simulink library "libFlightGearAnimation"  (R2020b)
settings: Solver=VariableStepAuto  StartTime=0.0  StopTime=10.0  RelTol=1e-3
undefined symbols (not defined in the file): outputs, Receive, Send, stepTime
libraries: aerolibconvert2 x3, aerolibfltsims x3, aerolibanimutils x1
settings Model: Creator=caatay  LastModifiedBy=caatay

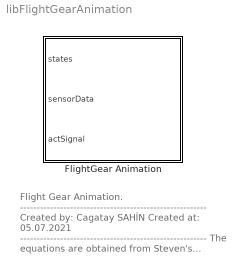
== system libFlightGearAnimation ==
  note: Flight Gear Animation.
      | --------------------------------------------------------
      | Created by: Cagatay SAHİN
      | Created at: 05.07.2021
      | --------------------------------------------------------
      | The equations are obtained from
      | Steven's textbook.
      | The reference book can be found in
      | "references folder".
      | --------------------------------------------------------
      | for question:
      | cagataysahin44@gmail.com
  FlightGear Animation : Subsystem  mask(Animation Model - Flight Gear Animation Model){stepTime=stepTime}
      mask prompts: stepTime "Step Sİze for each Step"
      mask help: Animation of aircraft's at whole simulation. That block use, states sensor data, actuator signals.
      mask Help:
      | This block is used for animate aircraft's motion in whole simulation.
      | --------------------------------------------------------------------------------------------------------------------------------------------------
      | Input of the function:
      | 	states: State Information
      | 	Sensor Data: Sensor Information.
      | 	Actuator Signal: Actuator Information
      | --------------------------------------------------------------------------------------------------------------------------------------------------
      | for question: "cagataysahin44@gmail.com"
      mask Display:
      | port_label('input',1,'states','texmode','on');
      | port_label('input',2,'sensorData','texmode','on');
      | port_label('input',3,'actSignal','texmode','on');

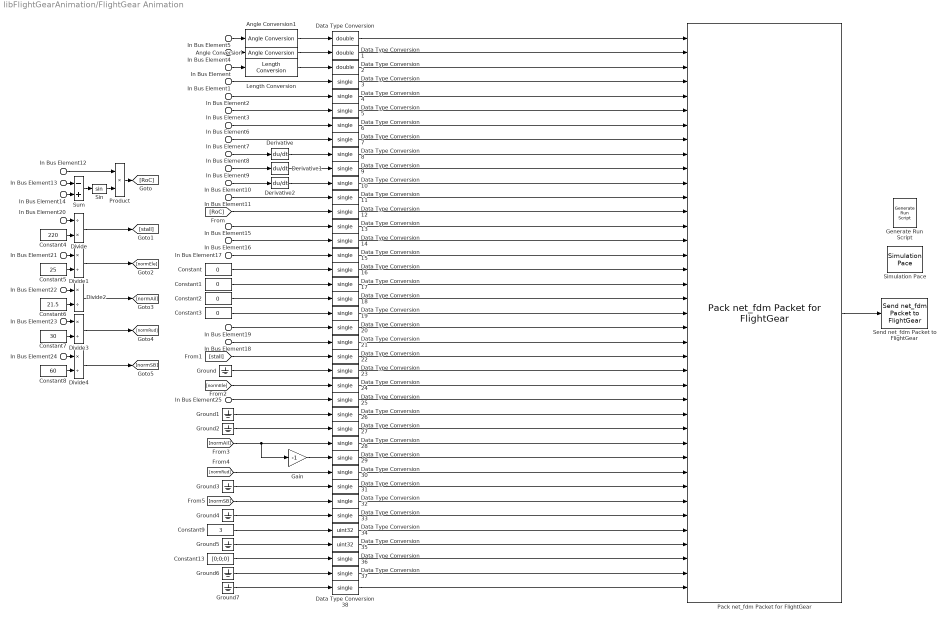
== system libFlightGearAnimation/FlightGear Animation ==
  In Bus Element : Inport  PortName=states  Element=z_e
  In Bus Element1 : Inport  PortName=states  Element=phi
  In Bus Element8 : Inport  PortName=states  Element=phi
  In Bus Element2 : Inport  PortName=states  Element=theta
  In Bus Element9 : Inport  PortName=states  Element=theta
  In Bus Element14 : Inport  PortName=states  Element=theta
  In Bus Element3 : Inport  PortName=states  Element=psi
  In Bus Element10 : Inport  PortName=states  Element=psi
  In Bus Element6 : Inport  PortName=states  Element=alpha
  In Bus Element13 : Inport  PortName=states  Element=alpha
  In Bus Element7 : Inport  PortName=states  Element=beta
  In Bus Element12 : Inport  PortName=states  Element=tas
  In Bus Element20 : Inport  PortName=states  Element=tas
  In Bus Element4 : Inport  Port=2  PortName=sensorData  Element=lat
  In Bus Element5 : Inport  Port=2  PortName=sensorData  Element=long
  In Bus Element11 : Inport  Port=2  PortName=sensorData  Element=ias
  In Bus Element15 : Inport  Port=2  PortName=sensorData  Element=u
  In Bus Element16 : Inport  Port=2  PortName=sensorData  Element=v
  In Bus Element17 : Inport  Port=2  PortName=sensorData  Element=w
  In Bus Element18 : Inport  Port=2  PortName=sensorData  Element=aN
  In Bus Element19 : Inport  Port=2  PortName=sensorData  Element=aY
  In Bus Element21 : Inport  Port=3  PortName=actSignal  Element=ele
  In Bus Element25 : Inport  Port=3  PortName=actSignal  Element=ele
  In Bus Element22 : Inport  Port=3  PortName=actSignal  Element=ail
  In Bus Element23 : Inport  Port=3  PortName=actSignal  Element=rud
  In Bus Element24 : Inport  Port=3  PortName=actSignal  Element=sb
  Angle Conversion : aerolibconvert2/Angle Conversion  IU=deg  OU=rad
  Angle Conversion1 : aerolibconvert2/Angle Conversion  IU=deg  OU=rad
  Constant{,1..3} (4 alike) : Constant  Value=0
  Constant13 : Constant  Value=[0;0;0]
  Constant4 : Constant  Value=220
  Constant5 : Constant  Value=25
  Constant6 : Constant  Value=21.5
  Constant7 : Constant  Value=30
  Constant8 : Constant  Value=60
  Constant9 : Constant  Value=3
  Data Type Conversion : DataTypeConversion  OutDataTypeStr=double
  Data Type Conversion1 : DataTypeConversion  OutDataTypeStr=double
  Data Type Conversion{3..33,36..38} (34 alike) : DataTypeConversion  OutDataTypeStr=single
  Data Type Conversion2 : DataTypeConversion  OutDataTypeStr=double
  Data Type Conversion34 : DataTypeConversion  OutDataTypeStr=uint32
  Data Type Conversion35 : DataTypeConversion  OutDataTypeStr=uint32
  Derivative : Derivative
  Derivative1 : Derivative
  Derivative2 : Derivative
  Divide : Product  Inputs=/*
  Divide{1..4} (4 alike) : Product  Inputs=*/
  Gain : Gain  Gain=-1
  Generate Run Script : aerolibfltsims/Generate Run Script  Architecture=Win64  dataFlow=Send-Receive  GeometryModelName=f16  AirportId=LTAE  RunwayId=03  InitialAltitude=outputs.trim.states.z_e  InitialHeading=outputs.trim.states.psi*180/pi  OffsetDistance=0  OffsetAzimuth=0  InstallScenery=on  DisableShaders=off  OriginAddress=127.0.0.1  DestinationPort=5502  OriginPort=5505  LocalAddress=127.0.0.1  OutputFileName=runfg.bat  FlightGearBaseDirectory=C:\Program Files\FlightGear
  Ground{,1..7} (8 alike) : Ground
  Length Conversion : aerolibconvert2/Length Conversion  IU=ft  OU=m
  Pack net_fdm Packet for FlightGear : aerolibfltsims/Pack net_fdm Packet for FlightGear  FlightGearVersion=v2019.1  ShowPositionAttitudeInputs=on  ShowVelocityAccelerationInputs=on  ShowControlSurfacePositionInputs=on  ShowEngineFuelInputs=off  ShowLandingGearInputs=on  ShowEnvironmentInputs=off  SampleTime=stepTime  packetVersion=24
      settings: SourceProductBaseCode=AE
  Product : Product
  Send net_fdm Packet to FlightGear : aerolibfltsims/Send net_fdm Packet to FlightGear  DestinationIpAddress=127.0.0.1  DestinationPort=5502  LocalIpPort=-1  varLen=off  SampleTime=stepTime
      settings: SourceProductBaseCode=AE
  Simulation Pace : aerolibanimutils/Simulation Pace  SimulationPace=1.5  SleepMode=Auto  OutputPaceError=off  SampleTime=stepTime
  Sin : Trigonometry
  Sum : Sum  Inputs=-+
  wires:
  Pack net_fdm Packet for FlightGear/1 -> Send net_fdm Packet to FlightGear/1
  In Bus Element/1 -> Length Conversion/1
  In Bus Element4/1 -> Angle Conversion/1
  Angle Conversion/1 -> Data Type Conversion1/1
  Angle Conversion1/1 -> Data Type Conversion/1
  In Bus Element5/1 -> Angle Conversion1/1
  Length Conversion/1 -> Data Type Conversion2/1
  Data Type Conversion/1 -> Pack net_fdm Packet for FlightGear/1
  Data Type Conversion1/1 -> Pack net_fdm Packet for FlightGear/2
  Data Type Conversion2/1 -> Pack net_fdm Packet for FlightGear/3
  Data Type Conversion5/1 -> Pack net_fdm Packet for FlightGear/6
  Data Type Conversion4/1 -> Pack net_fdm Packet for FlightGear/5
  Data Type Conversion3/1 -> Pack net_fdm Packet for FlightGear/4
  In Bus Element1/1 -> Data Type Conversion3/1
  In Bus Element2/1 -> Data Type Conversion4/1
  In Bus Element3/1 -> Data Type Conversion5/1
  In Bus Element6/1 -> Data Type Conversion6/1
  Data Type Conversion6/1 -> Pack net_fdm Packet for FlightGear/7
  In Bus Element7/1 -> Data Type Conversion7/1
  Data Type Conversion7/1 -> Pack net_fdm Packet for FlightGear/8
  In Bus Element10/1 -> Derivative2/1
  In Bus Element9/1 -> Derivative1/1
  In Bus Element8/1 -> Derivative/1
  Derivative/1 -> Data Type Conversion8/1
  Derivative2/1 -> Data Type Conversion10/1
  Derivative1/1 -> Data Type Conversion9/1
  Data Type Conversion8/1 -> Pack net_fdm Packet for FlightGear/9
  Data Type Conversion9/1 -> Pack net_fdm Packet for FlightGear/10
  Data Type Conversion10/1 -> Pack net_fdm Packet for FlightGear/11
  In Bus Element11/1 -> Data Type Conversion11/1
  Data Type Conversion11/1 -> Pack net_fdm Packet for FlightGear/12
  In Bus Element12/1 -> Product/1
  In Bus Element14/1 -> Sum/2
  In Bus Element13/1 -> Sum/1
  Sum/1 -> Sin/1
  Sin/1 -> Product/2
  Product/1 -> [RoC]
  [RoC] -> Data Type Conversion12/1
  Data Type Conversion12/1 -> Pack net_fdm Packet for FlightGear/13
  Data Type Conversion15/1 -> Pack net_fdm Packet for FlightGear/16
  In Bus Element17/1 -> Data Type Conversion15/1
  In Bus Element16/1 -> Data Type Conversion14/1
  Data Type Conversion14/1 -> Pack net_fdm Packet for FlightGear/15
  Data Type Conversion13/1 -> Pack net_fdm Packet for FlightGear/14
  In Bus Element15/1 -> Data Type Conversion13/1
  Data Type Conversion16/1 -> Pack net_fdm Packet for FlightGear/17
  Constant/1 -> Data Type Conversion16/1
  Data Type Conversion17/1 -> Pack net_fdm Packet for FlightGear/18
  Data Type Conversion18/1 -> Pack net_fdm Packet for FlightGear/19
  Constant2/1 -> Data Type Conversion18/1
  Constant1/1 -> Data Type Conversion17/1
  Constant3/1 -> Data Type Conversion19/1
  Data Type Conversion19/1 -> Pack net_fdm Packet for FlightGear/20
  In Bus Element18/1 -> Data Type Conversion21/1
  In Bus Element19/1 -> Data Type Conversion20/1
  Data Type Conversion20/1 -> Pack net_fdm Packet for FlightGear/21
  Data Type Conversion21/1 -> Pack net_fdm Packet for FlightGear/22
  Constant4/1 -> Divide/2
  In Bus Element20/1 -> Divide/1
  Divide/1 -> [stall]
  [stall] -> Data Type Conversion22/1
  Data Type Conversion22/1 -> Pack net_fdm Packet for FlightGear/23
  Data Type Conversion23/1 -> Pack net_fdm Packet for FlightGear/24
  Ground/1 -> Data Type Conversion23/1
  In Bus Element21/1 -> Divide1/1
  Constant5/1 -> Divide1/2
  Divide1/1 -> [normEle]
  In Bus Element22/1 -> Divide2/1
  Divide2/1 -> [normAil]
  Constant6/1 -> Divide2/2
  In Bus Element23/1 -> Divide3/1
  Constant7/1 -> Divide3/2
  Divide3/1 -> [normRud]
  Constant8/1 -> Divide4/2
  In Bus Element24/1 -> Divide4/1
  Divide4/1 -> [normSB]
  [normEle] -> Data Type Conversion24/1
  Data Type Conversion24/1 -> Pack net_fdm Packet for FlightGear/25
  In Bus Element25/1 -> Data Type Conversion25/1
  Data Type Conversion25/1 -> Pack net_fdm Packet for FlightGear/26
  Data Type Conversion27/1 -> Pack net_fdm Packet for FlightGear/28
  Data Type Conversion26/1 -> Pack net_fdm Packet for FlightGear/27
  Ground1/1 -> Data Type Conversion26/1
  Ground2/1 -> Data Type Conversion27/1
  [normAil] -> Gain/1, Data Type Conversion28/1
  Gain/1 -> Data Type Conversion29/1
  Data Type Conversion28/1 -> Pack net_fdm Packet for FlightGear/29
  Data Type Conversion29/1 -> Pack net_fdm Packet for FlightGear/30
  Data Type Conversion30/1 -> Pack net_fdm Packet for FlightGear/31
  [normRud] -> Data Type Conversion30/1
  Data Type Conversion32/1 -> Pack net_fdm Packet for FlightGear/33
  [normSB] -> Data Type Conversion32/1
  Data Type Conversion33/1 -> Pack net_fdm Packet for FlightGear/34
  Data Type Conversion31/1 -> Pack net_fdm Packet for FlightGear/32
  Ground3/1 -> Data Type Conversion31/1
  Ground4/1 -> Data Type Conversion33/1
  Constant9/1 -> Data Type Conversion34/1
  Data Type Conversion34/1 -> Pack net_fdm Packet for FlightGear/35
  Data Type Conversion35/1 -> Pack net_fdm Packet for FlightGear/36
  Ground5/1 -> Data Type Conversion35/1
  Data Type Conversion36/1 -> Pack net_fdm Packet for FlightGear/37
  Constant13/1 -> Data Type Conversion36/1
  Ground7/1 -> Data Type Conversion38/1
  Ground6/1 -> Data Type Conversion37/1
  Data Type Conversion37/1 -> Pack net_fdm Packet for FlightGear/38
  Data Type Conversion38/1 -> Pack net_fdm Packet for FlightGear/39
